simulink model "final_test"  (R2017a)
settings: Solver=VariableStepAuto  StartTime=0.0  StopTime=10.0  RelTol=1e-3
settings Model: Creator=ashwi  LastModifiedBy=ashwi

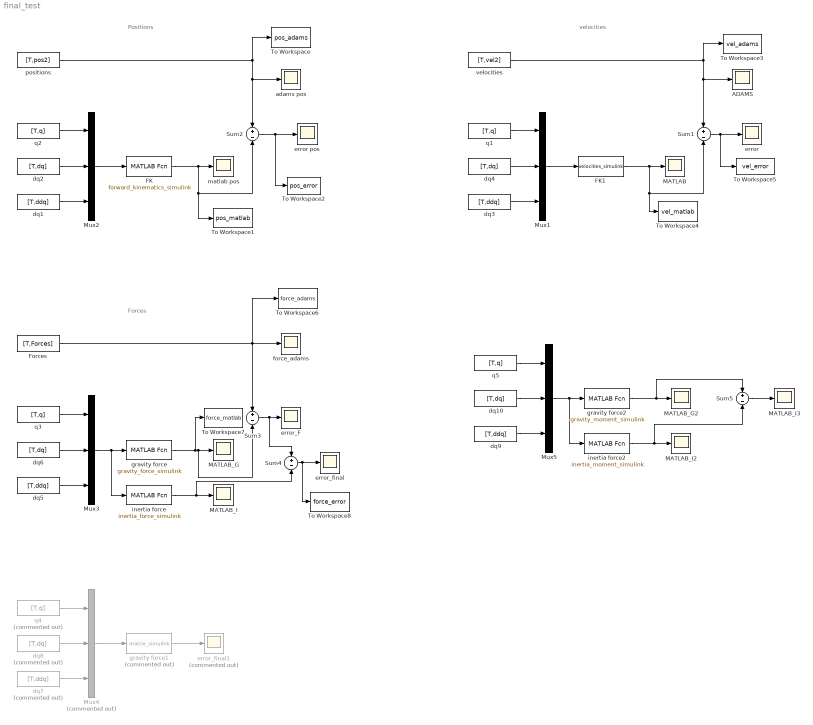
== system final_test ==
  note: Positions
  note: velocities
  note: Forces
  ADAMS : Scope
  FK : MATLABFcn  MATLABFcn=forward_kinematics_simulink
  FK1 : MATLABFcn  MATLABFcn=velocities_simulink
  Forces : FromWorkspace  VariableName=[T,Forces]  SampleTime=0
  MATLAB : Scope
  MATLAB_G : Scope
  MATLAB_G2 : Scope
  MATLAB_I : Scope
  MATLAB_I2 : Scope
  MATLAB_I3 : Scope
  Mux{1..3,5} (4 alike) : Mux  Inputs=3
  Mux4 : Mux  Commented=on  Inputs=3
  Sum{1..5} (5 alike) : Sum  Inputs=+-
  To Workspace : ToWorkspace  VariableName=pos_adams  SaveFormat=Timeseries  SampleTime=-1
  To Workspace1 : ToWorkspace  VariableName=pos_matlab  SaveFormat=Timeseries  SampleTime=-1
  To Workspace2 : ToWorkspace  VariableName=pos_error  SaveFormat=Timeseries  SampleTime=-1
  To Workspace3 : ToWorkspace  VariableName=vel_adams  SaveFormat=Timeseries  SampleTime=-1
  To Workspace4 : ToWorkspace  VariableName=vel_matlab  SaveFormat=Timeseries  SampleTime=-1
  To Workspace5 : ToWorkspace  VariableName=vel_error  SaveFormat=Timeseries  SampleTime=-1
  To Workspace6 : ToWorkspace  VariableName=force_adams  SaveFormat=Timeseries  SampleTime=-1
  To Workspace7 : ToWorkspace  VariableName=force_matlab  SaveFormat=Timeseries  SampleTime=-1
  To Workspace8 : ToWorkspace  VariableName=force_error  SaveFormat=Timeseries  SampleTime=-1
  adams pos : Scope
  dq{1,3,5,9} (4 alike) : FromWorkspace  VariableName=[T,ddq]  SampleTime=0
  dq{2,4,6,10} (4 alike) : FromWorkspace  VariableName=[T,dq]  SampleTime=0
  dq7 : FromWorkspace  Commented=on  VariableName=[T,ddq]  SampleTime=0
  dq8 : FromWorkspace  Commented=on  VariableName=[T,dq]  SampleTime=0
  error : Scope
  error pos : Scope
  error_F : Scope
  error_final : Scope
  error_final1 : Scope  Commented=on
  force_adams : Scope
  gravity force : MATLABFcn  MATLABFcn=gravity_force_simulink
  gravity force1 : MATLABFcn  Commented=on  MATLABFcn=matrix_simulink
  gravity force2 : MATLABFcn  MATLABFcn=gravity_moment_simulink
  inertia force : MATLABFcn  MATLABFcn=inertia_force_simulink
  inertia force2 : MATLABFcn  MATLABFcn=inertia_moment_simulink
  matlab pos : Scope
  positions : FromWorkspace  VariableName=[T,pos2]  SampleTime=0
  q{1..3,5} (4 alike) : FromWorkspace  VariableName=[T,q]  SampleTime=0
  q4 : FromWorkspace  Commented=on  VariableName=[T,q]  SampleTime=0
  velocities : FromWorkspace  VariableName=[T,vel2]  SampleTime=0
  wires:
  q2/1 -> Mux2/1
  positions/1 -> Sum2/1, adams pos/1, To Workspace/1
  Sum2/1 -> To Workspace2/1, error pos/1
  dq2/1 -> Mux2/2
  dq1/1 -> Mux2/3
  Mux2/1 -> FK/1
  FK/1 -> To Workspace1/1, Sum2/2, matlab pos/1
  velocities/1 -> To Workspace3/1, Sum1/1, ADAMS/1
  FK1/1 -> To Workspace4/1, Sum1/2, MATLAB/1
  Mux1/1 -> FK1/1
  q1/1 -> Mux1/1
  dq4/1 -> Mux1/2
  Sum1/1 -> To Workspace5/1, error/1
  dq3/1 -> Mux1/3
  Forces/1 -> To Workspace6/1, Sum3/1, force_adams/1
  gravity force/1 -> To Workspace7/1, Sum3/2, MATLAB_G/1
  Mux3/1 -> inertia force/1, gravity force/1
  q3/1 -> Mux3/1
  dq6/1 -> Mux3/2
  Sum3/1 -> Sum4/1, error_F/1
  dq5/1 -> Mux3/3
  inertia force/1 -> Sum4/2, MATLAB_I/1
  Sum4/1 -> To Workspace8/1, error_final/1
  gravity force1/1 -> error_final1/1
  Mux4/1 -> gravity force1/1
  dq7/1 -> Mux4/3
  q4/1 -> Mux4/1
  dq8/1 -> Mux4/2
  inertia force2/1 -> Sum5/2, MATLAB_I2/1
  q5/1 -> Mux5/1
  gravity force2/1 -> Sum5/1, MATLAB_G2/1
  dq9/1 -> Mux5/3
  Mux5/1 -> inertia force2/1, gravity force2/1
  dq10/1 -> Mux5/2
  Sum5/1 -> MATLAB_I3/1
